simulink library "libBusSerialize"  (R2015a)
settings: Solver=ode45  StartTime=0.0  StopTime=10.0  RelTol=1e-3
undefined symbols (not defined in the file): BusSerialize, macaddr, mxpcnetworkconfig, RigInfo, SimulinkParameter_TestParamPulse, SimulinkParameter_TestParamToggle, SimulinkParameter_TunableConditions, SimulinkParameter_TunableNextTrialId, SimulinkParameter_TunableTaskControl
libraries: simulink x5, xpcethernetlib x3, xpcnetworkbufferlib x2, xpcrtudplib x1
(part 2 of 2)

== matlab function libBusSerialize/Trigger Buffer/Active This Timestamp ==
  data: input input size=bufferSize; inputLen input uint32 size=1; buffer output size=bufferSize; lastTimestamp input; currentTimestamp input size=1; len output uint32 size=1
function [buffer, len]   = clearIfNewTimestamp(input, inputLen, lastTimestamp, currentTimestamp)
%#codegen

if lastTimestamp == currentTimestamp
    buffer = input;
    len = inputLen;
else
    buffer = [];
    len = cast(0, class(inputLen));
end

== matlab function libBusSerialize/Trigger Buffer/Triggered Append to Buffer Each Tick/MATLAB Function ==
  data: input input; buffer output size=bufferSize; timestamp input; len output uint32 size=1; bufferSize parameter size=1
function [buffer, len] = bufferEachTick(input, timestamp, bufferSize)
%#codegen

persistent pBuffer;
persistent pLastTimestamp;

coder.varsize('pBuffer', bufferSize, true);

clear = uint8(0);

% initialize persistents
if isempty(pBuffer) || isempty(pLastTimestamp)
    clear = uint8(1);
    pLastTimestamp = timestamp;
end

% determine if this is a new tick and reset the output if it is
if pLastTimestamp ~= timestamp
    pLastTimestamp = timestamp;
    clear = uint8(1);
end

if clear
    pBuffer = input(:);
elseif numel(pBuffer) == 0
    pBuffer = input(:);
elseif numel(pBuffer) + numel(input) < bufferSize
    pBuffer = [pBuffer; input(:)];
end

buffer = pBuffer;
len = uint32(numel(buffer));

== matlab function libBusSerialize/Unit-Delay Bus Memory/ToFixed ==
  data: in input; out output size=bufferSize; bufferSize parameter size=1
function out = variableToFixed(in, bufferSize)
%#codegen

out = zeros(bufferSize, 1, 'uint8'); %#ok<ZEROLIKE>

for i = 1:numel(in)
    if i > bufferSize
        break;
    end
    out(i) = in(i);
end

== matlab function libBusSerialize/Convert Variable to Fixed ==
  data: in input; out output size=bufferSize; bufferSize parameter size=1
function out = variableToFixed(in, bufferSize)
%#codegen

out = zeros(bufferSize, 1, 'uint8'); %#ok<ZEROLIKE>

for i = 1:numel(in)
    if i > bufferSize
        break;
    end
    out(i) = in(i);
end

== matlab function libBusSerialize/Unit-Delay Bus Memory/Deserialize ==
  data: bytes input; bus output Bus: RigOutputBus size=1; receivedInvalid output uint8 size=1
function [bus, receivedInvalid] = deserializeWithMemory(bytes)

%#codegen



    % cache input so we only deserialize when input changes

    persistent pBytes;

    if isempty(pBytes)

        pBytes = bytes;

        inChanged = uint8(1);

    elseif ~isequal(pBytes, bytes)

        pBytes = bytes;

        inChanged = uint8(1);

    else

        inChanged = uint8(0);

    end

    

    persistent pInvalid;

    if isempty(pInvalid)

        pInvalid = uint8(0);

    end



    % external cached output

    persistent pBusOut;

    if isempty(pBusOut)

        pBusOut = initializeBus_RigOutputBus();

    end



    % handle deserialization if changed

    if inChanged

        [tempBus, valid] = deserializeBus_RigOutputBus(bytes);

        if valid

            pBusOut = tempBus;

            pInvalid = uint8(0);

        else

            pInvalid = uint8(1);

        end

    end

         

    bus = pBusOut;

    receivedInvalid = pInvalid;

end

== matlab function libBusSerialize/Unit-Delay Bus Memory/Serialize ==
  data: busIn input Bus: RigOutputBus size=1; bytes output uint8 size=173164
function bytes = serialize(busIn)

%#codegen 



    bytes = serializeBus_RigOutputBus(busIn);



end

== matlab function libBusSerialize/Initialize Bus ==
  data: bus output Bus: TestBus size=1
function bus = initialize_TestBus()

%#codegen 



    bus = initializeBus_TestBus();



end

== matlab function libBusSerialize/Tunable Parameter Pulse Switch/Deserialize Parameter ==
  data: valAsDouble input double; value output uint8 size=[1 1]; update output uint8 size=1
function [value, update] = deserializeParameter(valAsDouble)
%#codegen

valAsBytes = typecast(valAsDouble, 'uint8');

% check for whether counter has been incremented
thisCounter = valAsBytes(1);
persistent pLastCounter;
if isempty(pLastCounter)
    pLastCounter = thisCounter;
end
if pLastCounter ~= thisCounter
    update = uint8(1);
    pLastCounter = thisCounter;
else
    update = uint8(0);
end

% typecast and reshape the value
if update ~= uint8(0)
    value = reshape(typecast(valAsBytes(double(2):double(2)), 'uint8'), [1 1]);
else
    value = uint8(0);
end

== matlab function libBusSerialize/Tunable Parameter Toggle Switch/Deserialize Parameter ==
  data: valAsDouble input double; value output uint8 size=[1 1]; update output uint8 size=1
function [value, update] = deserializeParameter(valAsDouble)
%#codegen

valAsBytes = typecast(valAsDouble, 'uint8');

% check for whether counter has been incremented
thisCounter = valAsBytes(1);
persistent pLastCounter;
if isempty(pLastCounter)
    pLastCounter = thisCounter;
end
if pLastCounter ~= thisCounter
    update = uint8(1);
    pLastCounter = thisCounter;
else
    update = uint8(0);
end

% typecast and reshape the value
value = reshape(typecast(valAsBytes(double(2):double(2)), 'uint8'), [1 1]);

== matlab function libBusSerialize/Serialized Bus Tunable Parameter/Deserialize Bus Parameter ==
  data: valAsDouble input double; bus output Bus: TaskControlBus size=1; update output uint8 size=1; allowPending input uint8 size=1; receivedInvalid output uint8 size=1
function [bus, update, receivedInvalid] = deserializeBusParameter(valAsDouble, allowPending)
%#codegen

    % typecast to bytes
    valAsBytes = typecast(valAsDouble, 'uint8');

    % use the first byte as updateCounter, check for whether counter has been incremented
    thisCounter = valAsBytes(1);
    persistent pLastCounter;
    if isempty(pLastCounter)
        pLastCounter = thisCounter;
    end
    if pLastCounter ~= thisCounter
        recvUpdate = uint8(1);
        pLastCounter = thisCounter;
    else
        recvUpdate = uint8(0);
    end
    startOffset = 2;

    % external cached output for when allowPending 
    persistent pBusOut;
    if isempty(pBusOut)
        pBusOut = initializeBus_TaskControlBus();
    end

    % parse incoming bytes if allowing updates
    receivedInvalid = uint8(0);
    if allowPending
        [bus, valid] = deserializeBus_TaskControlBus(valAsBytes, startOffset);
        if valid
            % update internal cache
            pBusOut = bus;
        else
            % don't update internal cache, output internal cache
            bus = pBusOut;
            receivedInvalid = uint8(1);
            recvUpdate = uint8(0);
        end
    else
        bus = pBusOut;
    end

    % track whether we have a pending update
    persistent pPending;
    if isempty(pPending), pPending = uint8(0); end
    if recvUpdate
        if allowPending
            % update goes out immediately
            update = uint8(1);
            pPending = uint8(0);
        else
            % queue pending update
            update = uint8(0);
            pPending = uint8(1);
        end
    else
        if allowPending
            % release pending
            update = pPending;
            pPending = uint8(0);
        else
            % do nothing
            update = uint8(0);
        end
    end

    % reset fields marked with .resetImmediately immediately after update
    if ~update
        bus.giveFreeJuice = uint8(0);
        bus.resetConditionBlock = uint8(0);

    end
end

== matlab function libBusSerialize/Convert Fixed to Variable ==
  data: in input; out output size=bufferSize; N input size=1; bufferSize parameter size=1
function out = fixedToVariable(in, N, bufferSize)
%#codegen

if N == 0
    out = zeros(0, 1, class(in)); %#ok<ZEROLIKE>
elseif N > bufferSize
    out = in;
else
    out = in(1:N);
end

== matlab function libBusSerialize/Tunable Serialized Conditions Array/Deserialize Parameter ==
  data: valAsDouble input double; value output uint8 size=109377; update output uint8 size=1
function [value, update] = deserializeParameter(valAsDouble)
%#codegen

valAsBytes = typecast(valAsDouble, 'uint8');

% check for whether counter has been incremented
thisCounter = valAsBytes(1);
persistent pLastCounter;
if isempty(pLastCounter)
    pLastCounter = thisCounter;
end
if pLastCounter ~= thisCounter
    update = uint8(1);
    pLastCounter = thisCounter;
else
    update = uint8(0);
end

% typecast and reshape the value
value = reshape(typecast(valAsBytes(double(2):double(109378)), 'uint8'), [109377 1]);
